simulink model "Problem_4week2"  (R2020a)
settings: Solver=VariableStepAuto  StartTime=0.0  StopTime=10.0  RelTol=1e-3
model workspace (MAT data in the model file):
  J = Simulink.Parameter
  J.Value = 3.2284e-06
  J.DataType = 'auto'
  J.Dimensions = [1 1]
  K = Simulink.Parameter
  K.Value = 0.0274
  K.DataType = 'auto'
  K.Dimensions = [1 1]
  L = Simulink.Parameter
  L.Value = 2.75e-06
  L.DataType = 'auto'
  L.Dimensions = [1 1]
  R = Simulink.Parameter
  R.Value = 4
  R.DataType = 'auto'
  R.Dimensions = [1 1]
  b = Simulink.Parameter
  b.Value = 3.5077e-06
  b.DataType = 'auto'
  b.Dimensions = [1 1]
  kd = Simulink.Parameter
  kd.Value = 0.139068731322
  kd.DataType = 'auto'
  kd.Dimensions = [1 1]
  ki = Simulink.Parameter
  ki.Value = 523.29550805
  ki.DataType = 'auto'
  ki.Dimensions = [1 1]
  kp = Simulink.Parameter
  kp.Value = 17.36824987
  kp.DataType = 'auto'
  kp.Dimensions = [1 1]
settings Model: Creator=hp  LastModifiedBy=hp

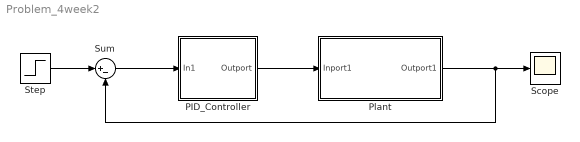
== system Problem_4week2 ==
  PID_Controller : Subsystem
  Plant : Subsystem
  Scope : Scope
  Step : Step  SampleTime=0
  Sum : Sum  Inputs=|+-
  wires:
  Sum/1 -> PID_Controller/1(In1)
  PID_Controller/1(Outport) -> Plant/1(Inport1)
  Plant/1(Outport1) -> Sum/2, Scope/1
  Step/1 -> Sum/1

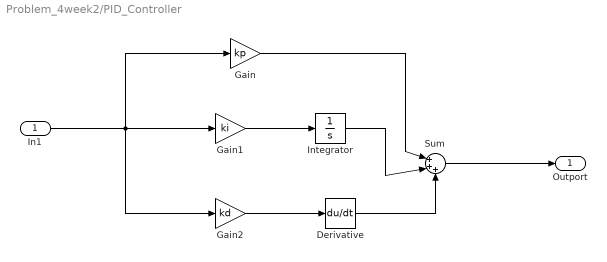
== system Problem_4week2/PID_Controller ==
  In1 : Inport
  Derivative : Derivative
  Gain : Gain  Gain=kp
  Gain1 : Gain  Gain=ki
  Gain2 : Gain  Gain=kd
  Integrator : Integrator
  Sum : Sum  Inputs=|+++
  Outport : Outport
  wires:
  Gain/1 -> Sum/1
  In1/1 -> Gain2/1, Gain/1, Gain1/1
  Gain1/1 -> Integrator/1
  Integrator/1 -> Sum/2
  Derivative/1 -> Sum/3
  Gain2/1 -> Derivative/1
  Sum/1 -> Outport/1

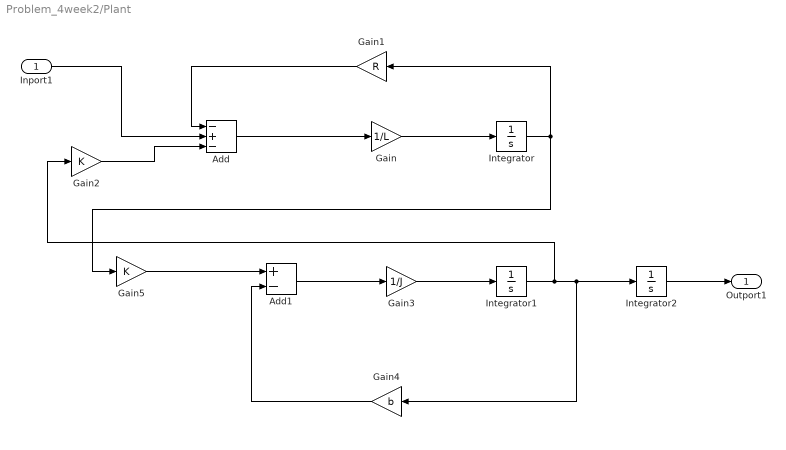
== system Problem_4week2/Plant ==
  Inport1 : Inport
  Add : Sum  Inputs=-+-
  Add1 : Sum  Inputs=+-
  Gain : Gain  Gain=1/L
  Gain1 : Gain  Gain=R
  Gain2 : Gain  Gain=K
  Gain3 : Gain  Gain=1/J
  Gain4 : Gain  Gain=b
  Gain5 : Gain  Gain=K
  Integrator : Integrator
  Integrator1 : Integrator
  Integrator2 : Integrator
  Outport1 : Outport
  wires:
  Integrator1/1 -> Gain2/1, Gain4/1, Integrator2/1
  Add1/1 -> Gain3/1
  Gain2/1 -> Add/3
  Gain5/1 -> Add1/1
  Inport1/1 -> Add/2
  Gain3/1 -> Integrator1/1
  Add/1 -> Gain/1
  Integrator/1 -> Gain5/1, Gain1/1
  Gain4/1 -> Add1/2
  Gain1/1 -> Add/1
  Gain/1 -> Integrator/1
  Integrator2/1 -> Outport1/1
